simulink library "SVPWM_Lib"  (R2023a)
settings: Solver=VariableStepAuto  StartTime=0.0  StopTime=10.0  RelTol=1e-3
undefined symbols (not defined in the file): Ts
settings Model: Creator=HP  LastModifiedBy=HP

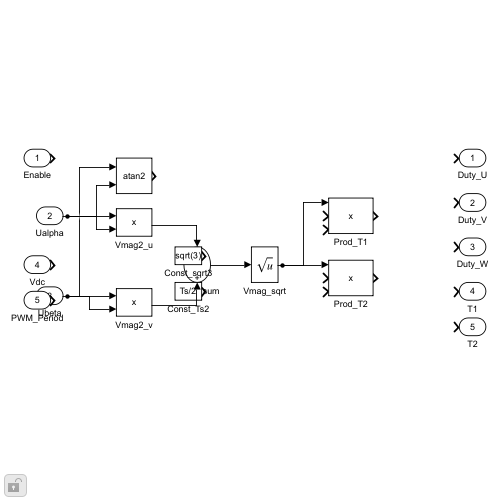
[thumbnail: Simulink's stored preview of the top-level diagram]
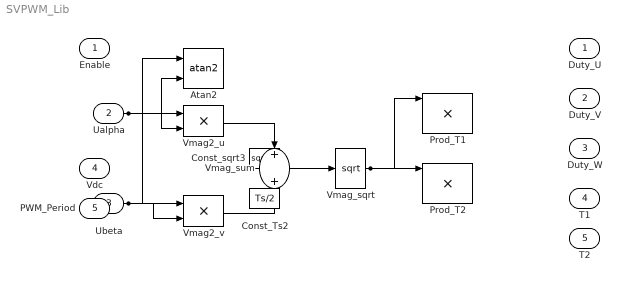
== system SVPWM_Lib ==
  Enable : Inport
  Ualpha : Inport  Port=2
  Ubeta : Inport  Port=3
  Vdc : Inport  Port=4
  PWM_Period : Inport  Port=5
  Atan2 : Trigonometry  Operator=atan2
  Const_Ts2 : Constant  Value=Ts/2
  Const_sqrt3 : Constant  Value=sqrt(3)
  Prod_T1 : Product  Inputs=***
  Prod_T2 : Product  Inputs=***
  Vmag2_u : Product  Inputs=**
  Vmag2_v : Product  Inputs=**
  Vmag_sqrt : Sqrt
  Vmag_sum : Sum
  Duty_U : Outport
  Duty_V : Outport  Port=2
  Duty_W : Outport  Port=3
  T1 : Outport  Port=4
  T2 : Outport  Port=5
  wires:
  Ubeta/1 -> Vmag2_v/2, Vmag2_v/1, Atan2/1
  Ualpha/1 -> Vmag2_u/2, Atan2/2, Vmag2_u/1
  Vmag2_u/1 -> Vmag_sum/1
  Vmag2_v/1 -> Vmag_sum/2
  Vmag_sum/1 -> Vmag_sqrt/1
  Vmag_sqrt/1 -> Prod_T1/1, Prod_T2/1
